simulink model "PMDCMotor"  (R2018a)
settings: Solver=ode45  StartTime=0.0  StopTime=.5  MaxStep=1e-3  RelTol=1e-4  AbsTol=1e-4  EnableMultiTasking=on
values from neighbouring files (symbols this model uses):
  Dm = .1209/615    (= 0.000196585365854)    [PMDCMotorparam.m]
  J = .0044    (= 0.0044)    [PMDCMotorparam.m]
  kt = .2198    (= 0.2198)    [PMDCMotorparam.m]
  Ra = .771    (= 0.771)    [PMDCMotorparam.m]
  Ta = La/Ra    (= 0.236057068742)    [PMDCMotorparam.m]
  Tm = .73    (= 0.73)    [PMDCMotorparam.m]
settings Model: Creator=Jurij  LastModifiedBy=Gianni
settings SolverCC: AutoScaleAbsTol=off
settings DataIOCC: LimitDataPoints=on  MaxDataPoints=10000  SaveFormat=Array  SignalLoggingSaveFormat=ModelDataLogs  SaveOutput=off  SaveState=on  StateSaveName=x  TimeSaveName=t  SignalLoggingName=sigsOut
settings OptimizationCC: LifeSpan=inf
settings DebuggingCC: SaveWithParameterizedLinksMsg=none  UnderspecifiedInitializationDetection=Classic  MergeDetectMultiDrivingBlocksExec=none  SignalResolutionControl=TryResolveAllWithWarning  MultiTaskDSMMsg=warning  MultiTaskCondExecSysMsg=none  SFUnexpectedBacktrackingDiag=warning  SFNoUnconditionalDefaultTransitionDiag=warning  SFExecutionAtInitializationDiag=none
settings HardwareCC: ProdBitPerPointer=32  ProdBitPerSizeT=32  ProdBitPerPtrDiffT=32  ProdLargestAtomicFloat=None  ProdIntDivRoundTo=Undefined  ProdEndianess=Unspecified  ProdWordSize=32  ProdHWDeviceType=32-bit Generic  TargetUnknown=on
settings ModelReferenceCC: PropagateSignalLabelsOutOfModel=off
settings CodeAppCC: StateflowObjectComments=on
settings GRTTargetCC: TargetLangStandard=C89/C90 (ANSI)  GeneratePreprocessorConditionals=Disable all  CombineOutputUpdateFcns=off  GRTInterface=on
settings ConfigComp: CovMetricSettings=dw  CovHtmlReporting=on  CovSaveCumulativeToWorkspaceVar=on  CovSaveSingleToWorkspaceVar=on  CovExternalEMLEnable=off

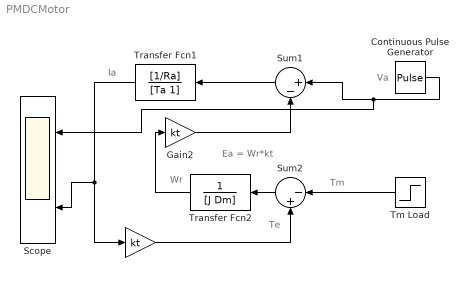
== system PMDCMotor ==
  note: Ia
  note: Ea = Wr*kt
  note: Wr
  note: Te
  note: Tm
  note: Va
  " " : Gain  Gain=kt
  Continuous Pulse Generator : DiscretePulseGenerator  PulseType=Time based  Amplitude=50  Period=1/10000  PulseWidth=50
  Gain2 : Gain  Gain=kt
  Scope : Scope  NumInputPorts=2
  Sum1 : Sum  Inputs=|+-  SaturateOnIntegerOverflow=on
  Sum2 : Sum  Inputs=|-+  SaturateOnIntegerOverflow=on
  Tm Load : Step  Time=0  Before=Tm  After=Tm  SampleTime=0
  Transfer Fcn1 : TransferFcn  Numerator=[1/Ra]  Denominator=[Ta 1]
  Transfer Fcn2 : TransferFcn  Denominator=[J Dm]
  wires:
  Sum1/1 -> Transfer Fcn1/1
  Transfer Fcn2/1 -> Gain2/1
  Gain2/1 -> Sum1/2
  Sum2/1 -> Transfer Fcn2/1
  Transfer Fcn1/1 -> " "/1, Scope/2
  " "/1 -> Sum2/2
  Continuous Pulse Generator/1 -> Scope/1, Sum1/1
  Tm Load/1 -> Sum2/1
